simulink model "servos_logics"  (R2018b)
settings: Solver=FixedStepAuto  StartTime=0.0  StopTime=inf  RelTol=1e-3  EnableMultiTasking=on
libraries: bbblueActuatorLib x8, simulink x2
settings Model: SimulationMode=external  ExtModeTrigDuration=100  Creator=Neal  LastModifiedBy=CHEI
settings SolverCC: PositivePriorityOrder=on
settings OptimizationCC: EnhancedBackFolding=on  PassReuseOutputArgsAs=Individual arguments  MaxStackSize=64  OptimizeBlockOrder=speed  DifferentSizesBufferReuse=on  OptimizationCustomize=off
settings DebuggingCC: ParameterTunabilityLossMsg=error
settings HardwareCC: ProdBitPerPointer=32  ProdBitPerSizeT=32  ProdBitPerPtrDiffT=32  ProdLargestAtomicInteger=Long  ProdLargestAtomicFloat=Double  ProdWordSize=32  ProdHWDeviceType=ARM Compatible->ARM Cortex
settings SFSimCC: MATLABDynamicMemAlloc=off
settings RTWCC: SystemTargetFile=ert.tlc  HardwareBoard=BeagleBone Blue  TLCOptions="-aInlineSetEventsForThisBaseRateFcn=TLC_FALSE -aSuppressMultiTaskScheduler=TLC_FALSE  -aRateBasedStepFcn=0"  TemplateMakefile=ert_default_tmf  GenerateReport=on  Toolchain=GNU GCC BeagleBone Blue  IncludeHyperlinkInReport=on  LaunchReport=on  GenerateTraceInfo=on  GenerateTraceReport=on  GenerateTraceReportSl=on  GenerateTraceReportSf=on  GenerateTraceReportEml=on
settings CodeAppCC: ForceParamTrailComments=on  IgnoreCustomStorageClasses=off  OperatorAnnotations=on  SimulinkDataObjDesc=on  SFDataObjDesc=on  InsertBlockDesc=on
settings ERTTargetCC: SupportVariableSizeSignals=on

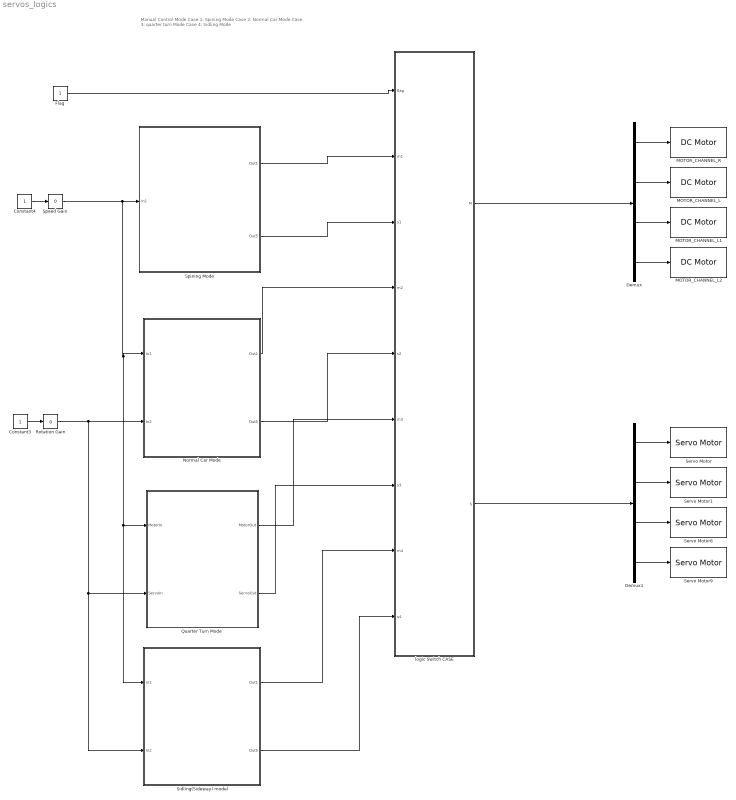
== system servos_logics ==
  note: Manual Control Mode
      |
      | Case 1: Spining Mode
      | Case 2: Normal Car Mode
      | Case 3: quarter turn Mode
      | Case 4: Sidling Mode
  Constant3 : Constant
  Constant4 : Constant
  Demux : Demux
  Demux1 : Demux
  Flag : Constant
  MOTOR_CHANNEL_L : bbblueActuatorLib/DC Motor  index=2  stopaction=Brake  SimulateUsing=Code generation
      settings: SourceProductName=Simulink Coder Support Package for BeagleBone Blue Hardware
  MOTOR_CHANNEL_L1 : bbblueActuatorLib/DC Motor  index=3  stopaction=Brake  SimulateUsing=Code generation
      settings: SourceProductName=Simulink Coder Support Package for BeagleBone Blue Hardware
  MOTOR_CHANNEL_L2 : bbblueActuatorLib/DC Motor  index=4  stopaction=Brake  SimulateUsing=Code generation
      settings: SourceProductName=Simulink Coder Support Package for BeagleBone Blue Hardware
  MOTOR_CHANNEL_R : bbblueActuatorLib/DC Motor  index=1  stopaction=Brake  SimulateUsing=Code generation
      settings: SourceProductName=Simulink Coder Support Package for BeagleBone Blue Hardware
  Normal Car Mode : Subsystem
  Quarter Turn Mode : Subsystem
  Rotation Gain : simulink/Math Operations/Slider Gain  gain=0  low=-0.45  high=0.45
  Servo Motor : bbblueActuatorLib/Servo Motor  channel=1  SimulateUsing=Code generation
      settings: SourceProductName=Simulink Coder Support Package for BeagleBone Blue Hardware
  Servo Motor1 : bbblueActuatorLib/Servo Motor  channel=2  SimulateUsing=Code generation
      settings: SourceProductName=Simulink Coder Support Package for BeagleBone Blue Hardware
  Servo Motor8 : bbblueActuatorLib/Servo Motor  channel=3  SimulateUsing=Code generation
      settings: SourceProductName=Simulink Coder Support Package for BeagleBone Blue Hardware
  Servo Motor9 : bbblueActuatorLib/Servo Motor  channel=4  SimulateUsing=Code generation
      settings: SourceProductName=Simulink Coder Support Package for BeagleBone Blue Hardware
  Sidling(Sideway) model : Subsystem
  Speed Gain : simulink/Math Operations/Slider Gain  gain=0  low=-1  high=1
  Spining Mode : Subsystem
  logic Switch CASE : MATLAB Function  TreatAsAtomicUnit=on
  wires:
  Constant4/1 -> Speed Gain/1
  Speed Gain/1 -> Sidling(Sideway) model/1(In1), Quarter Turn Mode/1(MotorIn), Normal Car Mode/1(In1), Spining Mode/1(In1)
  Demux/2 -> MOTOR_CHANNEL_L/1
  Demux/1 -> MOTOR_CHANNEL_R/1
  Demux/3 -> MOTOR_CHANNEL_L1/1
  Demux/4 -> MOTOR_CHANNEL_L2/1
  Demux1/1 -> Servo Motor/1
  Demux1/2 -> Servo Motor1/1
  Demux1/3 -> Servo Motor8/1
  Demux1/4 -> Servo Motor9/1
  Rotation Gain/1 -> Sidling(Sideway) model/2(In2), Quarter Turn Mode/2(ServoIn), Normal Car Mode/2(In2)
  Constant3/1 -> Rotation Gain/1
  Spining Mode/1(Out1) -> logic Switch CASE/2(m1)
  Spining Mode/2(Out5) -> logic Switch CASE/3(s1)
  Normal Car Mode/1(Out1) -> logic Switch CASE/4(m2)
  Normal Car Mode/2(Out5) -> logic Switch CASE/5(s2)
  logic Switch CASE/2(S) -> Demux1/1
  logic Switch CASE/1(M) -> Demux/1
  Flag/1 -> logic Switch CASE/1(flag)
  Sidling(Sideway) model/1(Out1) -> logic Switch CASE/8(m4)
  Sidling(Sideway) model/2(Out5) -> logic Switch CASE/9(s4)
  Quarter Turn Mode/1("MotorOut ") -> logic Switch CASE/6(m3)
  Quarter Turn Mode/2(ServoOut) -> logic Switch CASE/7(s3)

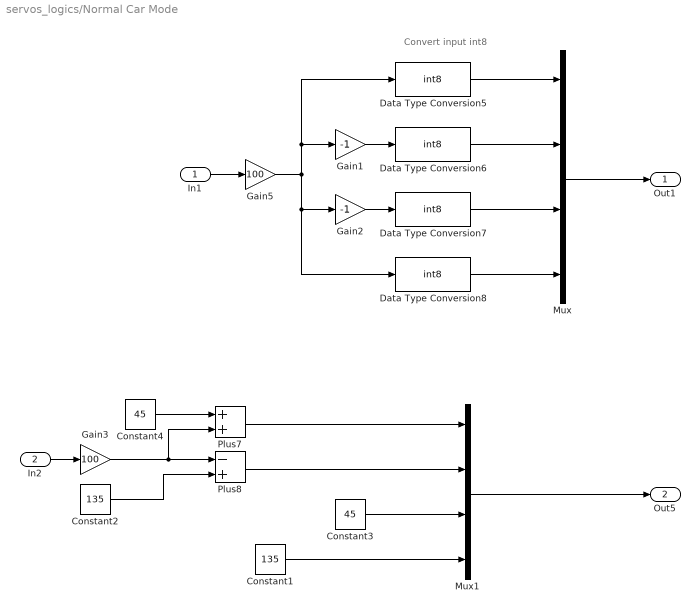
== system servos_logics/Normal Car Mode ==
  note: Convert input
      | int8
  In1 : Inport
  In2 : Inport  Port=2
  Constant1 : Constant  Value=135
  Constant2 : Constant  Value=135
  Constant3 : Constant  Value=45
  Constant4 : Constant  Value=45
  Data Type Conversion{5..8} (4 alike) : DataTypeConversion  OutDataTypeStr=int8  SaturateOnIntegerOverflow=on  RndMeth=Zero
  Gain1 : Gain  Gain=-1
  Gain2 : Gain  Gain=-1
  Gain3 : Gain  Gain=100
  Gain5 : Gain  Gain=100
  Mux : Mux
  Mux1 : Mux
  Plus7 : Sum
  Plus8 : Sum  Inputs=-+
  Out1 : Outport
  Out5 : Outport  Port=2
  wires:
  Gain5/1 -> Data Type Conversion5/1, Gain1/1, Gain2/1, Data Type Conversion8/1
  In1/1 -> Gain5/1
  Data Type Conversion5/1 -> Mux/1
  Data Type Conversion6/1 -> Mux/2
  Data Type Conversion7/1 -> Mux/3
  Data Type Conversion8/1 -> Mux/4
  Mux/1 -> Out1/1
  Mux1/1 -> Out5/1
  Gain1/1 -> Data Type Conversion6/1
  Gain2/1 -> Data Type Conversion7/1
  Constant3/1 -> Mux1/3
  Constant1/1 -> Mux1/4
  Constant4/1 -> Plus7/1
  Plus7/1 -> Mux1/1
  Plus8/1 -> Mux1/2
  In2/1 -> Gain3/1
  Constant2/1 -> Plus8/2
  Gain3/1 -> Plus7/2, Plus8/1

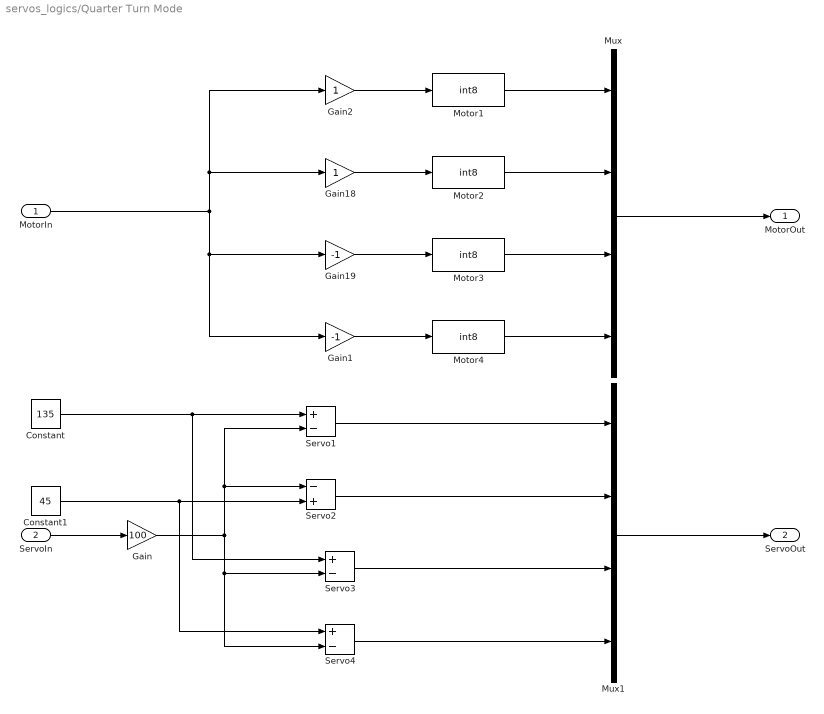
== system servos_logics/Quarter Turn Mode ==
  MotorIn : Inport
  ServoIn : Inport  Port=2
  Constant : Constant  Value=135
  Constant1 : Constant  Value=45
  Gain : Gain  Gain=100
  Gain1 : Gain  Gain=-1
  Gain18 : Gain
  Gain19 : Gain  Gain=-1
  Gain2 : Gain
  Motor{1..4} (4 alike) : DataTypeConversion  OutDataTypeStr=int8
  Mux : Mux
  Mux1 : Mux
  Servo1 : Sum  Inputs=+-
  Servo2 : Sum  Inputs=-+
  Servo3 : Sum  Inputs=+-
  "Servo4 " : Sum  Inputs=+-
  "MotorOut " : Outport
  ServoOut : Outport  Port=2
  wires:
  Gain19/1 -> Motor3/1
  Motor3/1 -> Mux/3
  Motor2/1 -> Mux/2
  Motor4/1 -> Mux/4
  MotorIn/1 -> Gain19/1, Gain1/1, Gain2/1, Gain18/1
  Gain18/1 -> Motor2/1
  Mux/1 -> "MotorOut "/1
  Motor1/1 -> Mux/1
  ServoIn/1 -> Gain/1
  Gain/1 -> "Servo4 "/2, Servo3/2, Servo1/2, Servo2/1
  Servo1/1 -> Mux1/1
  Mux1/1 -> ServoOut/1
  Constant1/1 -> "Servo4 "/1, Servo2/2
  Servo2/1 -> Mux1/2
  Constant/1 -> Servo3/1, Servo1/1
  "Servo4 "/1 -> Mux1/4
  Gain1/1 -> Motor4/1
  Gain2/1 -> Motor1/1
  Servo3/1 -> Mux1/3

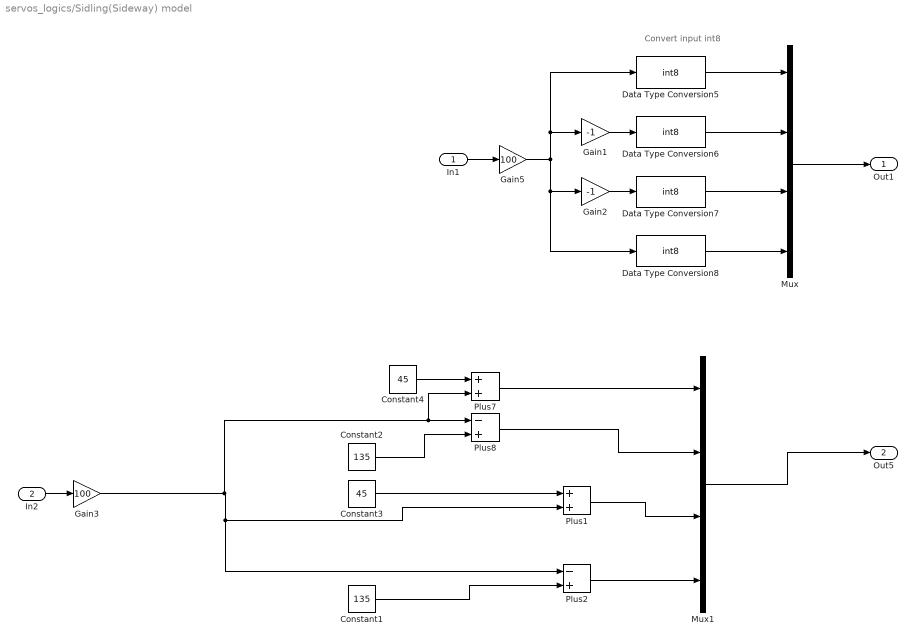
== system servos_logics/Sidling(Sideway) model ==
  note: Convert input
      | int8
  In1 : Inport
  In2 : Inport  Port=2
  Constant1 : Constant  Value=135
  Constant2 : Constant  Value=135
  Constant3 : Constant  Value=45
  Constant4 : Constant  Value=45
  Data Type Conversion{5..8} (4 alike) : DataTypeConversion  OutDataTypeStr=int8  SaturateOnIntegerOverflow=on  RndMeth=Zero
  Gain1 : Gain  Gain=-1
  Gain2 : Gain  Gain=-1
  Gain3 : Gain  Gain=100
  Gain5 : Gain  Gain=100
  Mux : Mux
  Mux1 : Mux
  Plus1 : Sum
  Plus2 : Sum  Inputs=-+
  Plus7 : Sum
  Plus8 : Sum  Inputs=-+
  Out1 : Outport
  Out5 : Outport  Port=2
  wires:
  Gain5/1 -> Data Type Conversion5/1, Gain1/1, Gain2/1, Data Type Conversion8/1
  In1/1 -> Gain5/1
  Data Type Conversion5/1 -> Mux/1
  Data Type Conversion6/1 -> Mux/2
  Data Type Conversion7/1 -> Mux/3
  Data Type Conversion8/1 -> Mux/4
  Mux/1 -> Out1/1
  Mux1/1 -> Out5/1
  Gain1/1 -> Data Type Conversion6/1
  Gain2/1 -> Data Type Conversion7/1
  Constant4/1 -> Plus7/1
  Plus7/1 -> Mux1/1
  Plus8/1 -> Mux1/2
  In2/1 -> Gain3/1
  Constant2/1 -> Plus8/2
  Constant3/1 -> Plus1/1
  Plus1/1 -> Mux1/3
  Plus2/1 -> Mux1/4
  Constant1/1 -> Plus2/2
  Gain3/1 -> Plus2/1, Plus1/2, Plus7/2, Plus8/1

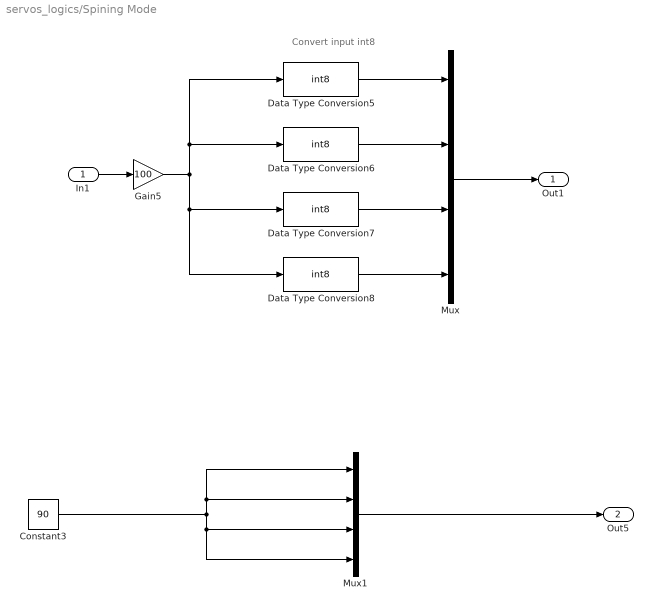
== system servos_logics/Spining Mode ==
  note: Convert input
      | int8
  In1 : Inport
  Constant3 : Constant  Value=90
  Data Type Conversion{5..8} (4 alike) : DataTypeConversion  OutDataTypeStr=int8  SaturateOnIntegerOverflow=on  RndMeth=Zero
  Gain5 : Gain  Gain=100
  Mux : Mux
  Mux1 : Mux
  Out1 : Outport
  Out5 : Outport  Port=2
  wires:
  Gain5/1 -> Data Type Conversion5/1, Data Type Conversion6/1, Data Type Conversion7/1, Data Type Conversion8/1
  In1/1 -> Gain5/1
  Data Type Conversion5/1 -> Mux/1
  Data Type Conversion6/1 -> Mux/2
  Data Type Conversion7/1 -> Mux/3
  Data Type Conversion8/1 -> Mux/4
  Mux/1 -> Out1/1
  Constant3/1 -> Mux1/2, Mux1/1, Mux1/3, Mux1/4
  Mux1/1 -> Out5/1

== matlab function servos_logics/logic Switch CASE ==
  data: flag input; M output; m1 input; s1 input; m2 input; s2 input; m3 input; s3 input; S output; m4 input; s4 input
function [M,S]= fcn(flag,m1,s1,m2,s2,m3,s3,m4,s4)
if flag == 1
    M = m1;
    S = s1;
elseif  flag == 2
    M = m2;
    S = s2;
elseif flag ==3
    
    M = m3;
    S = s3;
else 
    M = m4;
    S = s4;
    end


end
